simulink model "simulacion"  (R2020a)
settings: Solver=VariableStepAuto  StartTime=0.0  StopTime=0.6  RelTol=1e-3
values from neighbouring files (symbols this model uses):
  denominador1 = [1,-L]    [lab10.m]
  denominador2 = [1,-L]    [lab10.m]
  denominador3 = [2,-2]    [lab10.m]
  f = 10    [lab10.m]
  numerador1 = [1-L,0]    [lab10.m]
  numerador2 = [L,-L]    [lab10.m]
  numerador3 = [1e-3,1e-3]    [lab10.m]
  Ts = 0.001    [lab10.m]
settings Model: Creator=isaac  LastModifiedBy=isaac

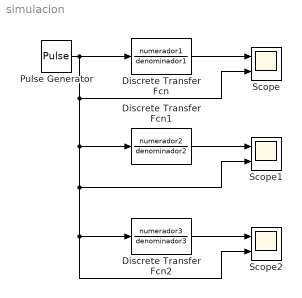
== system simulacion ==
  Discrete Transfer Fcn : DiscreteTransferFcn  Numerator=numerador1  Denominator=denominador1  SampleTime=Ts
  Discrete Transfer Fcn1 : DiscreteTransferFcn  Numerator=numerador2  Denominator=denominador2  SampleTime=Ts
  Discrete Transfer Fcn2 : DiscreteTransferFcn  Numerator=numerador3  Denominator=denominador3  SampleTime=Ts
  Pulse Generator : DiscretePulseGenerator  PulseType=Time based  Amplitude=3  Period=1/f  PulseWidth=50
  Scope : Scope  NumInputPorts=2
  Scope1 : Scope  NumInputPorts=2
  Scope2 : Scope  NumInputPorts=2
  wires:
  Discrete Transfer Fcn/1 -> Scope/1
  Discrete Transfer Fcn1/1 -> Scope1/1
  Pulse Generator/1 -> Scope1/2, Scope2/2, Discrete Transfer Fcn2/1, Discrete Transfer Fcn1/1, Scope/2, Discrete Transfer Fcn/1
  Discrete Transfer Fcn2/1 -> Scope2/1
